simulink model "SMTestBusModel"  (R2024b)
settings: Solver=FixedStepAuto  StartTime=0.0  StopTime=inf  FixedStep=0.1  RelTol=1e-3
undefined symbols (not defined in the file or in its folder): libBusSerialize, Serialize
settings Model: Creator=aillar  LastModifiedBy=kev
settings DebuggingCC: UnitsInconsistencyMsg=none

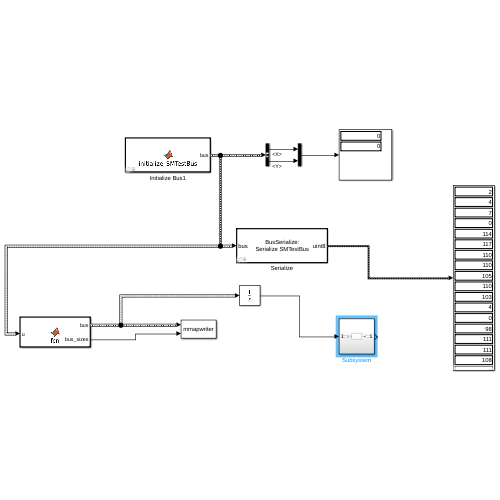
[thumbnail: Simulink's stored preview of the top-level diagram]
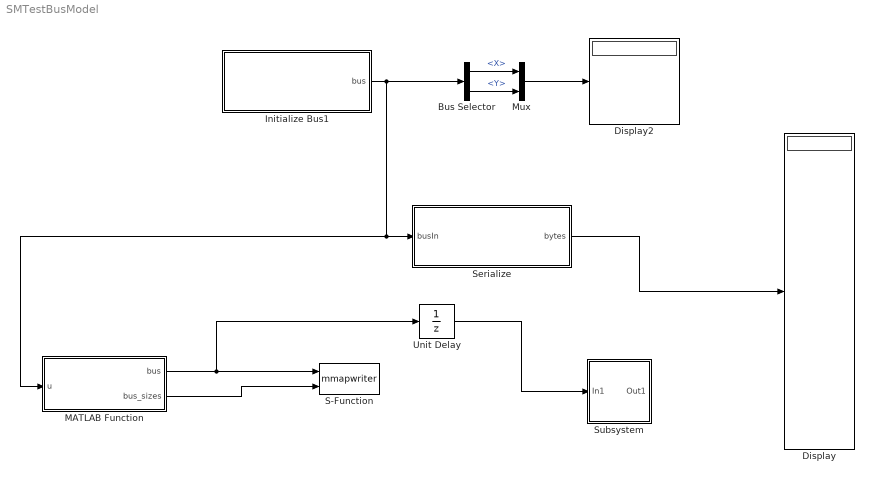
== system SMTestBusModel ==
  Bus Selector : BusSelector  OutputSignals=analog.X,analog.Y
  Display : Display
  Display2 : Display
  Initialize Bus1 : MATLAB Function  AncestorBlock=libBusSerialize/Initialize Bus  TreatAsAtomicUnit=on  mask(Initialize Bus Block){busType=Bus: SMTestBus}
      mask prompts: busType "Bus Type:"
      mask help: This block simply wraps an initializeBus_BusName() function and is useful for debugging where bus inputs are required. It acts essentially like a ground source for bus types.
      mask init:
      | BusSerialize.maskInitializeBusBlockUpdate(gcb);
  MATLAB Function : MATLAB Function  TreatAsAtomicUnit=on
  Mux : Mux  Inputs=2
  S-Function : S-Function  FunctionName=mmapwriter  Parameters=SMTestBus, 'Testing'  SFunctionDeploymentMode=off  EnableBusSupport=off
  Serialize : MATLAB Function  AncestorBlock=libBusSerialize/Serialize  TreatAsAtomicUnit=on  mask(BusSerialize: serialize block){busType=Bus: SMTestBus}
      mask prompts: busType "Bus Type"
      mask help: Select the bus type below to serialize.
      mask init:
      | BusSerialize.maskSerializeBlockUpdate(gcb)
  Subsystem : Subsystem
  Unit Delay : UnitDelay  SampleTime=-1  HasFrameUpgradeWarning=on
  wires:
  Mux/1 -> Display2/1
  Initialize Bus1/1(bus) -> MATLAB Function/1(u), Serialize/1(busIn), Bus Selector/1
  Bus Selector/1 -> Mux/1  "<X>"
  Bus Selector/2 -> Mux/2  "<Y>"
  Serialize/1(bytes) -> Display/1
  MATLAB Function/1(bus) -> Unit Delay/1, S-Function/1
  MATLAB Function/2(bus_sizes) -> S-Function/2
  Unit Delay/1 -> Subsystem/1(In1)

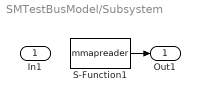
== system SMTestBusModel/Subsystem ==
  In1 : Inport
  S-Function1 : S-Function  FunctionName=mmapreader  Parameters=Testing  SFunctionDeploymentMode=off  EnableBusSupport=off
  Out1 : Outport
  wires:
  S-Function1/1 -> Out1/1

== matlab function SMTestBusModel/MATLAB Function ==
  data: u input Bus: SMTestBus; bus output Bus: SMTestBus; bus_sizes output int32
function [bus, bus_sizes]  = fcn(u)
    flat_dims = zeros(getLen(u), 2, 'int32');
    counter = ones(1);
    [flat_dims, counter] = getDims(u, flat_dims, counter);
    disp(flat_dims);
    bus_sizes = flat_dims;
    bus = u;
end

function len = getLen(bus)
    fields = fieldnames(bus);
    len = 0;
    for iF = 1:numel(fields)
        field = fields{iF};
        if isfield(bus, field)
            value = bus.(field);
            if isa(value, 'struct')
                len = len + getLen(value);
            else
                len = len + 1;
            end
        end
    end
end

function [flat_dims, counter] = getDims(bus, flat_dims, counter)
    fields = fieldnames(bus);
    for iF = 1:numel(fields)
        field = fields{iF};
        if isfield(bus, field)
            value = bus.(field);
            if isa(value, 'struct')
                [flat_dims, counter] = getDims(value, flat_dims, counter);
            else
                flat_dims(counter(1), :) = size(value);
                disp(field);
                disp(value);
                counter(1) = counter(1) + 1;
            end
        end
    end
end

== matlab function SMTestBusModel/Initialize Bus1 ==
  data: bus output Bus: SMTestBus size=1
function bus = initialize_SMTestBus()
%#codegen 

    bus = initializeBus_SMTestBus();

end

== matlab function SMTestBusModel/Serialize ==
  data: busIn input Bus: SMTestBus size=1; bytes output uint8 size=67404
function bytes = serialize(busIn)
%#codegen 

    bytes = serializeBus_SMTestBus(busIn);

end
